simulink model "adder_r12"  (Simulink 4.0)
settings: Solver=FixedStepDiscrete  StartTime=0.0  StopTime=10.0  RelTol=1e-3
settings Model: Creator=sofronis  LastModifiedBy=sofronis  AlgebraicLoopMsg=error  BooleanDataType=on

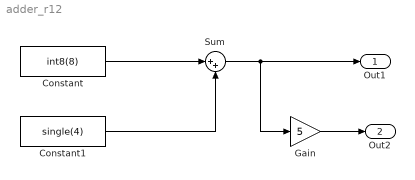
== system adder_r12 ==
  Constant : Constant  Value=int8(8)
  Constant1 : Constant  Value=single(4)
  Gain : Gain  Gain=5  Multiplication=Element-wise(K.*u)  SaturateOnIntegerOverflow=on
  Sum : Sum  Inputs=|++  SaturateOnIntegerOverflow=on
  Out1 : Outport  Port=1
  Out2 : Outport  Port=2
  wires:
  Constant/1 -> Sum/1
  Constant1/1 -> Sum/2
  Sum/1 -> Out1/1, Gain/1
  Gain/1 -> Out2/1
